simulink library "v2l"  (R2021b)
settings: Solver=VariableStepAuto  StartTime=0.0  StopTime=10.0  RelTol=1e-3
undefined symbols (not defined in the file): AV2L_SOCV2LLimit_X_pct, C_TASK_1000MS_S, ENUM_OBCV2LSTA_WORKING, ENUM_REQOBCEXTRV2L_EXTERNALDISCHRG, ENUM_REQOBCINTRV2L_INTERNALDISCHRG, ENUM_REQV2LIVIDISCHRG_DISCHRG, ENUM_REQV2LIVIDISCHRG_OFF, FALSE, KV2L_HVBattSOCLimit_pct, KV2L_HVPOGrpCheckOvrd_flg, KV2L_HVPOGrplowerLimit_pct, KV2L_HVPOGrpUpperLimit_pct, KV2L_OBCACCurrInfLimit_A, KV2L_SOCV2LSetLimit_pct, MV2L_SOCV2LLimit_Y_pct
libraries: hcu_lib x3, nmm x1, FVT_lib x1
settings Model: Creator=FVT23010  LastModifiedBy=FVT23010

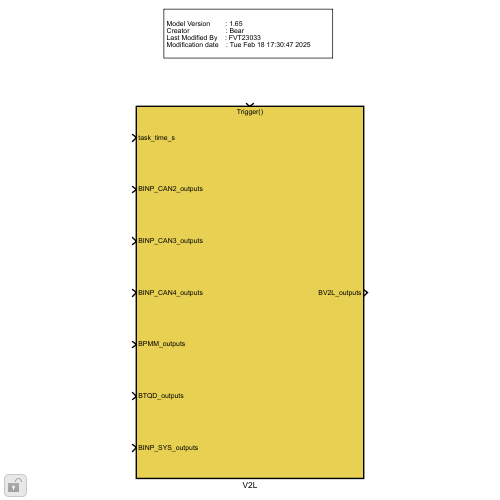
[thumbnail: Simulink's stored preview of the top-level diagram]
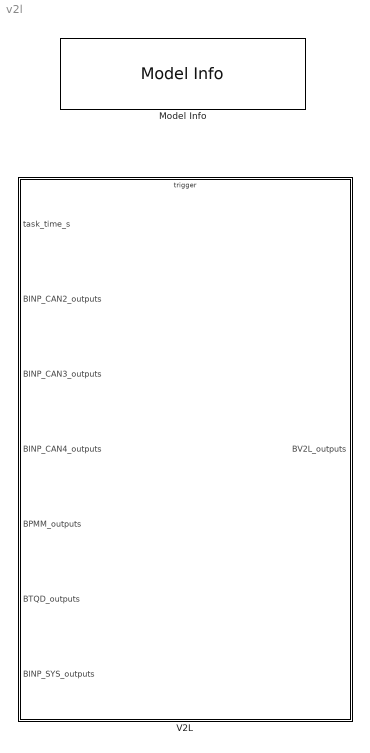
== system v2l ==
  Model Info : nmm/Model Info  InitialBlockCM=None  BlockCM=None  Frame=on  DisplayStringWithTags=|  HorizontalTextAlignment=Left  LeftAlignmentValue=0.02  SourceBlockDiagram=pmm  TagMaxNumber=20
      | Model Version        : %<ModelVersion>
      | Creator                   : Bear
      | Last Modified By    : %<LastModifiedBy>
      | Modification date    : %<LastModificationDate>
  V2L : Subsystem
      settings: RTWSystemCode=Nonreusable function  RTWFcnNameOpts=Use subsystem name  RTWFileNameOpts=Use subsystem name

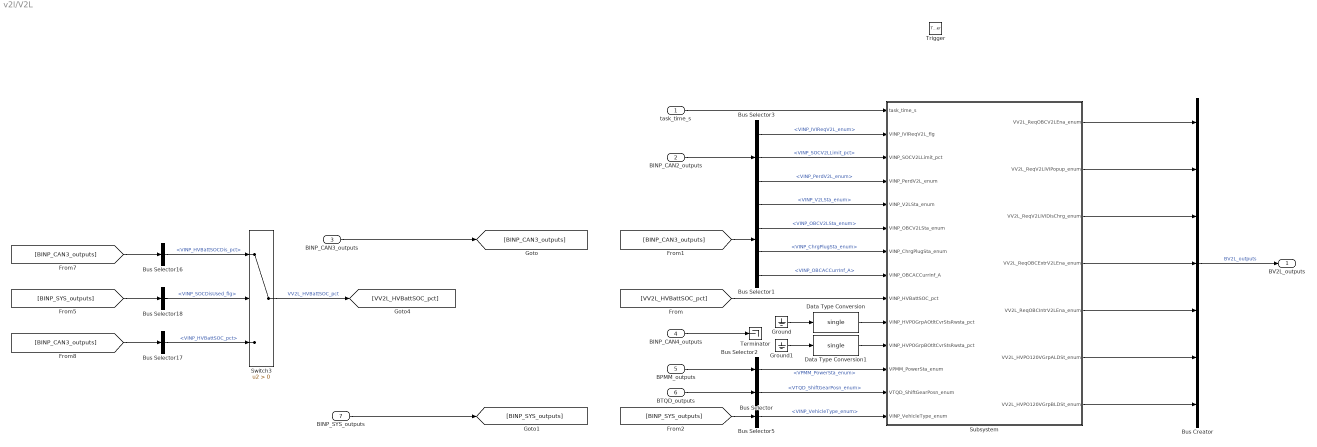
== system v2l/V2L ==
  task_time_s : Inport
  BINP_CAN2_outputs : Inport  Port=2  OutDataTypeStr=Bus: BINP_CAN2_outputs
  BINP_CAN3_outputs : Inport  Port=3  OutDataTypeStr=Bus: BINP_CAN3_outputs
  BINP_CAN4_outputs : Inport  Port=4  OutDataTypeStr=Bus: BINP_CAN4_outputs
  BPMM_outputs : Inport  Port=5  OutDataTypeStr=Bus: BPMM_outputs
  BTQD_outputs : Inport  Port=6  OutDataTypeStr=Bus: BTQD_outputs
  BINP_SYS_outputs : Inport  Port=7  OutDataTypeStr=Bus: BINP_SYS_outputs
  Trigger : TriggerPort  TriggerType=function-call  VariantControl=(inherit)  PortDimensions=1
  Bus Creator : BusCreator  Inputs=7  OutDataTypeStr=Bus: BV2L_outputs  NonVirtualBus=on
  Bus Selector : BusSelector  OutputSignals=VTQD_ShiftGearPosn_enum
  Bus Selector1 : BusSelector  OutputSignals=VINP_V2LSta_enum,VINP_OBCV2LSta_enum,VINP_ChrgPlugSta_enum,VINP_OBCACCurrInf_A
  Bus Selector16 : BusSelector  OutputSignals=VINP_HVBattSOCDis_pct
  Bus Selector17 : BusSelector  OutputSignals=VINP_HVBattSOC_pct
  Bus Selector18 : BusSelector  OutputSignals=VINP_SOCDisUsed_flg
  Bus Selector2 : BusSelector  OutputSignals=VPMM_PowerSta_enum
  Bus Selector3 : BusSelector  OutputSignals=VINP_IVIReqV2L_enum,VINP_SOCV2LLimit_pct,VINP_PerdV2L_enum
  Bus Selector5 : BusSelector  OutputSignals=VINP_VehicleType_enum
  Data Type Conversion : DataTypeConversion  OutDataTypeStr=single
  Data Type Conversion1 : DataTypeConversion  OutDataTypeStr=single
  Ground : Ground
  Ground1 : Ground
  Subsystem : Subsystem
  Switch3 : Switch  Criteria=u2 > Threshold
  Terminator : Terminator
  BV2L_outputs : Outport  OutDataTypeStr=Bus: BV2L_outputs
  wires:
  BPMM_outputs/1 -> Bus Selector2/1
  BTQD_outputs/1 -> Bus Selector/1
  BINP_CAN2_outputs/1 -> Bus Selector3/1
  Bus Creator/1 -> BV2L_outputs/1  "BV2L_outputs"
  Bus Selector3/1 -> Subsystem/2(VINP_IVIReqV2L_flg)  "<VINP_IVIReqV2L_enum>"
  Bus Selector3/2 -> Subsystem/3(VINP_SOCV2LLimit_pct)  "<VINP_SOCV2LLimit_pct>"
  Bus Selector3/3 -> Subsystem/4(VINP_PerdV2L_enum)  "<VINP_PerdV2L_enum>"
  Bus Selector1/1 -> Subsystem/5(VINP_V2LSta_enum)  "<VINP_V2LSta_enum>"
  Bus Selector1/2 -> Subsystem/6(VINP_OBCV2LSta_enum)  "<VINP_OBCV2LSta_enum>"
  Bus Selector1/3 -> Subsystem/7(VINP_ChrgPlugSta_enum)  "<VINP_ChrgPlugSta_enum>"
  Bus Selector1/4 -> Subsystem/8(VINP_OBCACCurrInf_A)  "<VINP_OBCACCurrInf_A>"
  Bus Selector2/1 -> Subsystem/12(VPMM_PowerSta_enum)  "<VPMM_PowerSta_enum>"
  Bus Selector/1 -> Subsystem/13(VTQD_ShiftGearPosn_enum)  "<VTQD_ShiftGearPosn_enum>"
  task_time_s/1 -> Subsystem/1(task_time_s)
  Subsystem/1(VV2L_ReqOBCV2LEna_enum) -> Bus Creator/1
  Subsystem/2(VV2L_ReqV2LIVIPopup_enum) -> Bus Creator/2
  Subsystem/3(VV2L_ReqV2LIVIDisChrg_enum) -> Bus Creator/3
  Subsystem/4(VV2L_ReqOBCExtrV2LEna_enum) -> Bus Creator/4
  Subsystem/5(VV2L_ReqOBCIntrV2LEna_enum) -> Bus Creator/5
  Subsystem/6(VV2L_HVPO120VGrpALDSt_enum) -> Bus Creator/6
  Subsystem/7(VV2L_HVPO120VGrpBLDSt_enum) -> Bus Creator/7
  Bus Selector5/1 -> Subsystem/14(VINP_VehicleType_enum)  "<VINP_VehicleType_enum>"
  Bus Selector16/1 -> Switch3/1  "<VINP_HVBattSOCDis_pct>"
  [BINP_CAN3_outputs] -> Bus Selector16/1
  [BINP_CAN3_outputs] -> Bus Selector17/1
  Switch3/1 -> [VV2L_HVBattSOC_pct]  "VV2L_HVBattSOC_pct"
  [BINP_SYS_outputs] -> Bus Selector18/1
  Bus Selector17/1 -> Switch3/3  "<VINP_HVBattSOC_pct>"
  Bus Selector18/1 -> Switch3/2  "<VINP_SOCDisUsed_flg>"
  [VV2L_HVBattSOC_pct] -> Subsystem/9(VINP_HVBattSOC_pct)
  BINP_CAN3_outputs/1 -> [BINP_CAN3_outputs]
  [BINP_CAN3_outputs] -> Bus Selector1/1
  BINP_SYS_outputs/1 -> [BINP_SYS_outputs]
  [BINP_SYS_outputs] -> Bus Selector5/1
  BINP_CAN4_outputs/1 -> Terminator/1
  Ground/1 -> Data Type Conversion/1
  Data Type Conversion/1 -> Subsystem/10(VINP_HVPOGrpAOtltCvrStsRwsta_pct)
  Ground1/1 -> Data Type Conversion1/1
  Data Type Conversion1/1 -> Subsystem/11(VINP_HVPOGrpBOtltCvrStsRwsta_pct)

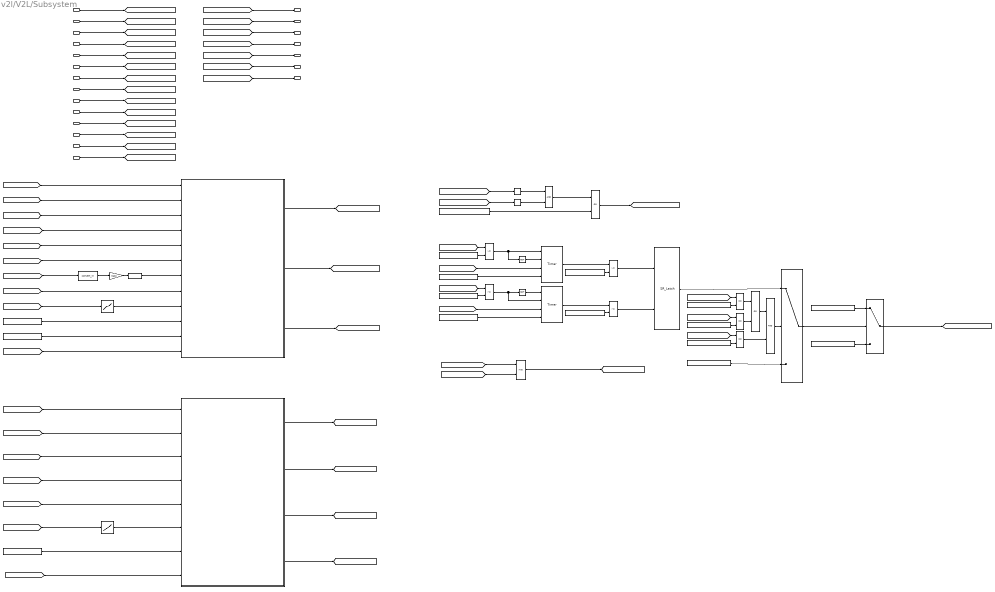
== system v2l/V2L/Subsystem ==
  task_time_s : Inport
  VINP_IVIReqV2L_flg : Inport  Port=2
  VINP_SOCV2LLimit_pct : Inport  Port=3
  VINP_PerdV2L_enum : Inport  Port=4
  VINP_V2LSta_enum : Inport  Port=5
  VINP_OBCV2LSta_enum : Inport  Port=6
  VINP_ChrgPlugSta_enum : Inport  Port=7
  VINP_OBCACCurrInf_A : Inport  Port=8
  VINP_HVBattSOC_pct : Inport  Port=9
  VINP_HVPOGrpAOtltCvrStsRwsta_pct : Inport  Port=10
  VINP_HVPOGrpBOtltCvrStsRwsta_pct : Inport  Port=11
  VPMM_PowerSta_enum : Inport  Port=12
  VTQD_ShiftGearPosn_enum : Inport  Port=13
  VINP_VehicleType_enum : Inport  Port=14
  1-D Lookup Table : Lookup_n-D  NumberOfTableDimensions=1  BreakpointsForDimension1=AV2L_SOCV2LLimit_X_pct  Table=MV2L_SOCV2LLimit_Y_pct  InternalRulePriority=Speed  RndMeth=Simplest  InputSameDT=on
  1-D Lookup Table1 : Lookup_n-D  NumberOfTableDimensions=1  BreakpointsForDimension1=AV2L_SOCV2LLimit_X_pct  Table=MV2L_SOCV2LLimit_Y_pct  InternalRulePriority=Speed  RndMeth=Simplest  InputSameDT=on
  Constant : Constant  Value=KV2L_HVBattSOCLimit_pct
  Constant1 : Constant  Value=KV2L_SOCV2LSetLimit_pct
  Constant10 : Constant  Value=ENUM_REQV2LIVIDISCHRG_OFF
  Constant11 : Constant  Value=ENUM_REQV2LIVIDISCHRG_DISCHRG
  Constant12 : Constant  Value=ENUM_REQOBCEXTRV2L_EXTERNALDISCHRG
  Constant13 : Constant  Value=ENUM_REQOBCINTRV2L_INTERNALDISCHRG
  Constant14 : Constant  Value=KV2L_HVPOGrpCheckOvrd_flg
  Constant15 : Constant  Value=ENUM_OBCV2LSTA_WORKING
  Constant2 : Constant  Value=KV2L_HVBattSOCLimit_pct
  Constant3 : Constant  Value=KV2L_OBCACCurrInfLimit_A
  Constant{4..5,7..8} (4 alike) : Constant  Value=C_TASK_1000MS_S
  Constant6 : Constant  Value=KV2L_OBCACCurrInfLimit_A
  Constant9 : Constant  Value=FALSE
  Data Type Conversion : DataTypeConversion  OutDataTypeStr=single
  External V2L : Stateflow chart  TreatAsAtomicUnit=on
      settings: PortSchema="{\"entries\":[{\"content\":{\"sides\":[{\"content\":{\"connectorIds\":[\"In1\",\"In2\",\"In3\",\"In4\",\"In5\",\"In6\",\"In7\",\"In8\",\"In9\",\"In10\",\"In11\",\"In12\"]},\"type\":\"ConnectorPlacement.EquallySpacedRectSide\",\"uuid\":\"45116e41-1dba-4e2c-ae04-6007bf1e0ef0\"},{\"content\":{\"connectorIds\":[\"Out1\",\"Out3\",\"Out2\"],\"side\":\"RIGHT\"},\"type\":\"ConnectorPlacement.EquallySpacedRectSide\",\"uuid\":\"1413f850-bb59-4483-bd31-f1fc97818d70\"},{\"content\":{\"connectorIds\":[],\"side\":\"TOP\"},\"type\":\"ConnectorPlacement.EquallySpacedRectSide\",\"uuid\":\"54439ff1-b412-4fc1-ba32-699466081697\"}]},\"type\":\"ConnectorPlacement.EquallySpacedConnector\",\"uuid\":\"a2cf914b-1bae-4478-a72c-e2494d61996c\"}],\"packageUris\":[\"http://schema.mathworks.com/mf0/Connector/R2020b\"],\"version\":\"1.0\"}"
  Gain : Gain  Gain=3600
  Internal V2L : Stateflow chart  TreatAsAtomicUnit=on
  Logical Operator : Logic  AllPortsSameDT=off  OutDataTypeStr=boolean
  Logical Operator1 : Logic  Operator=NOT  AllPortsSameDT=off  OutDataTypeStr=boolean
  Logical Operator2 : Logic  Operator=NOT  AllPortsSameDT=off  OutDataTypeStr=boolean
  Logical Operator3 : Logic  Operator=OR  AllPortsSameDT=off  OutDataTypeStr=boolean
  Logical Operator4 : Logic  AllPortsSameDT=off  OutDataTypeStr=boolean
  Logical Operator5 : Logic  Operator=OR  AllPortsSameDT=off  OutDataTypeStr=boolean
  MinMax : MinMax  Function=max  Inputs=2
  Relational Operator{,1..3} (4 alike) : RelationalOperator  OutDataTypeStr=boolean  RndMeth=Simplest
  Relational Operator4 : RelationalOperator  Operator===  OutDataTypeStr=boolean  RndMeth=Simplest
  Relational Operator5 : RelationalOperator  Operator===  OutDataTypeStr=boolean  RndMeth=Simplest
  Relational Operator6 : RelationalOperator  Operator===  OutDataTypeStr=boolean  RndMeth=Simplest
  Relay : Relay  OnSwitchValue=KV2L_HVPOGrpUpperLimit_pct  OffSwitchValue=KV2L_HVPOGrplowerLimit_pct
  Relay1 : Relay  OnSwitchValue=KV2L_HVPOGrpUpperLimit_pct  OffSwitchValue=KV2L_HVPOGrplowerLimit_pct
  SR_Latch : hcu_lib/Basic_Blocks/SR_Latch
  Switch : Switch  Criteria=u2 ~= 0
  Switch1 : Switch  Criteria=u2 ~= 0
  Timer : hcu_lib/Basic_Blocks/Timer
  Timer1 : hcu_lib/Basic_Blocks/Timer
  convert_in9 : FVT_lib/hal/convert_in  gain=0.5  offset=0.5
  VV2L_ReqOBCV2LEna_enum : Outport
  VV2L_ReqV2LIVIPopup_enum : Outport  Port=2
  VV2L_ReqV2LIVIDisChrg_enum : Outport  Port=3
  VV2L_ReqOBCExtrV2LEna_enum : Outport  Port=4
  VV2L_ReqOBCIntrV2LEna_enum : Outport  Port=5
  VV2L_HVPO120VGrpALDSt_enum : Outport  Port=6
  VV2L_HVPO120VGrpBLDSt_enum : Outport  Port=7
  wires:
  task_time_s/1 -> [task_time_s]
  [VV2L_ReqOBCExtrV2LEna_enum] -> VV2L_ReqOBCExtrV2LEna_enum/1
  [task_time_s] -> External V2L/1(task_time_s)
  Constant1/1 -> External V2L/11(KV2L_SOCV2LSetLimit_pct)
  External V2L/1(VV2L_ReqOBCExtrV2LEna_enum) -> [VV2L_ReqOBCExtrV2LEna_enum]
  VTQD_ShiftGearPosn_enum/1 -> [VTQD_ShiftGearPosn_enum]
  VINP_IVIReqV2L_flg/1 -> [VINP_IVIReqV2L_flg]
  VINP_SOCV2LLimit_pct/1 -> [VINP_SOCV2LLimit_pct]
  VINP_V2LSta_enum/1 -> [VINP_V2LSta_enum]
  VINP_OBCV2LSta_enum/1 -> [VINP_OBCV2LSta_enum]
  [VINP_HVBattSOC_pct] -> External V2L/6(VINP_HVBattSOC_pct)
  VINP_PerdV2L_enum/1 -> [VINP_PerdV2L_enum]
  [VINP_SOCV2LLimit_pct] -> 1-D Lookup Table/1
  VPMM_PowerSta_enum/1 -> [VPMM_PowerSta_enum]
  [VINP_IVIReqV2L_flg] -> External V2L/2(VINP_IVIReqV2L_flg)
  [VINP_V2LSta_enum] -> External V2L/5(VINP_V2LSta_enum)
  [VINP_OBCV2LSta_enum] -> External V2L/8(VINP_OBCV2LSta_enum)
  VINP_HVBattSOC_pct/1 -> [VINP_HVBattSOC_pct]
  [VPMM_PowerSta_enum] -> External V2L/3(VPMM_PowerSta_enum)
  Constant/1 -> External V2L/10(KV2L_HVBattSOCLimit_pct)
  [VV2L_ReqV2LIVIPopup_enum] -> VV2L_ReqV2LIVIPopup_enum/1
  [VTQD_ShiftGearPosn_enum] -> External V2L/4(VTQD_ShiftGearPosn_enum)
  Data Type Conversion/1 -> External V2L/7(VV2L_PerdV2LSet_s)  "VV2L_PerdV2LSet_s"
  Gain/1 -> Data Type Conversion/1
  [VINP_PerdV2L_enum] -> convert_in9/1
  convert_in9/1 -> Gain/1
  1-D Lookup Table/1 -> External V2L/9(VV2L_SOCV2LLimit_pct)  "VV2L_SOCV2LLimit_pct"
  Constant2/1 -> Internal V2L/7(KV2L_HVBattSOCLimit_pct)
  [VPMM_PowerSta_enum] -> Internal V2L/3(VPMM_PowerSta_enum)
  [VINP_OBCV2LSta_enum] -> Internal V2L/5(VINP_OBCV2LSta_enum)
  [VINP_SOCV2LLimit_pct] -> 1-D Lookup Table1/1
  [VINP_HVBattSOC_pct] -> Internal V2L/4(VINP_HVBattSOC_pct)
  VINP_ChrgPlugSta_enum/1 -> [VINP_ChrgPlugSta_enum]
  [VINP_ChrgPlugSta_enum] -> Internal V2L/1(VINP_ChrgPlugSta_enum)
  [VINP_HVPOGrpAOtltCvrStsRwsta_pct] -> Relay/1
  [VINP_HVPOGrpBOtltCvrStsRwsta_pct] -> Relay1/1
  Relay/1 -> Logical Operator/1
  Relay1/1 -> Logical Operator/2
  Logical Operator/1 -> Logical Operator5/1
  [VV2L_HVPOGrpCheck_flg] -> Internal V2L/2(VV2L_HVPOGrpCheck_flg)
  VINP_OBCACCurrInf_A/1 -> [VINP_OBCACCurrInf_A]
  [VINP_OBCACCurrInf_A] -> Relational Operator/1
  Constant3/1 -> Relational Operator/2
  Relational Operator/1 -> Logical Operator1/1, Timer/1
  Logical Operator1/1 -> Timer/2
  [task_time_s] -> Timer/3
  Constant4/1 -> Timer/4
  Timer/1 -> Relational Operator1/1
  Constant5/1 -> Relational Operator1/2
  Relational Operator1/1 -> SR_Latch/1
  Relational Operator3/1 -> SR_Latch/2
  Constant8/1 -> Relational Operator3/2
  Timer1/1 -> Relational Operator3/1
  Constant7/1 -> Timer1/4
  [task_time_s] -> Timer1/3
  Relational Operator2/1 -> Timer1/2, Logical Operator2/1
  Constant6/1 -> Relational Operator2/2
  [VINP_OBCACCurrInf_A] -> Relational Operator2/1
  Logical Operator2/1 -> Timer1/1
  SR_Latch/1 -> Switch/1
  Internal V2L/1(VV2L_ReqOBCIntrV2LEna_enum) -> [VV2L_ReqOBCIntrV2LEna_enum]
  [VV2L_ReqExtrV2LIVIPopup_enum] -> MinMax/1
  Internal V2L/4(VV2L_ReqIntrV2LIVIPopup_enum) -> [VV2L_ReqIntrV2LIVIPopup_enum]
  [VV2L_ReqIntrV2LIVIPopup_enum] -> MinMax/2
  MinMax/1 -> [VV2L_ReqV2LIVIPopup_enum]  "VV2L_ReqV2LIVIPopup_enum"
  Switch/1 -> Switch1/2
  [VV2L_ReqOBCExtrV2LEna_enum] -> Relational Operator4/1
  [VV2L_ReqOBCIntrV2LEna_enum] -> Relational Operator5/1
  Logical Operator3/1 -> Logical Operator4/1
  Constant9/1 -> Switch/3
  Internal V2L/3(VV2L_HVPO120VGrpBLDSt_enum) -> [VV2L_HVPO120VGrpBLDSt_enum]
  Internal V2L/2(VV2L_HVPO120VGrpALDSt_enum) -> [VV2L_HVPO120VGrpALDSt_enum]
  1-D Lookup Table1/1 -> Internal V2L/6(VV2L_SOCV2LLimit_pct)  "VV2L_SOCV2LLimit_pct"
  [VV2L_ReqOBCIntrV2LEna_enum] -> VV2L_ReqOBCIntrV2LEna_enum/1
  [VV2L_ReqV2LIVIDisChrg_enum] -> VV2L_ReqV2LIVIDisChrg_enum/1
  [VV2L_HVPO120VGrpALDSt_enum] -> VV2L_HVPO120VGrpALDSt_enum/1
  [VV2L_HVPO120VGrpBLDSt_enum] -> VV2L_HVPO120VGrpBLDSt_enum/1
  VINP_HVPOGrpAOtltCvrStsRwsta_pct/1 -> [VINP_HVPOGrpAOtltCvrStsRwsta_pct]
  VINP_HVPOGrpBOtltCvrStsRwsta_pct/1 -> [VINP_HVPOGrpBOtltCvrStsRwsta_pct]
  [VV2L_ReqOBCV2LEna_enum] -> VV2L_ReqOBCV2LEna_enum/1
  External V2L/2(VV2L_ReqExtrV2LIVIPopup_enum) -> [VV2L_ReqExtrV2LIVIPopup_enum]
  External V2L/3(VV2L_ReqOBCV2LEna_enum) -> [VV2L_ReqOBCV2LEna_enum]
  Constant10/1 -> Switch1/3
  Constant11/1 -> Switch1/1
  Switch1/1 -> [VV2L_ReqV2LIVIDisChrg_enum]  "VV2L_ReqV2LIVIDisChrg_enum"
  Logical Operator4/1 -> Switch/2
  [VINP_OBCV2LSta_enum] -> Relational Operator6/1
  Relational Operator4/1 -> Logical Operator3/1
  Relational Operator5/1 -> Logical Operator3/2
  Constant12/1 -> Relational Operator4/2
  Constant13/1 -> Relational Operator5/2
  Logical Operator5/1 -> [VV2L_HVPOGrpCheck_flg]  "VV2L_HVPOGrpCheck_flg"
  Constant14/1 -> Logical Operator5/2
  VINP_VehicleType_enum/1 -> [VINP_VehicleType_enum]
  [VINP_VehicleType_enum] -> Internal V2L/8(VINP_VehicleType_enum)
  [VINP_VehicleType_enum] -> External V2L/12(VINP_VehicleType_enum)
  Constant15/1 -> Relational Operator6/2
  Relational Operator6/1 -> Logical Operator4/2

== stateflow chart v2l/V2L/Subsystem/Internal V2L ==
  state V2L
    en:
    VV2L_ReqOBCIntrV2LEna_enum = ENUM_REQOBCINTRV2L_NOREQUEST;
    VV2L_ReqIntrV2LIVIPopup_enum = ENUM_REQV2LIVI_NOREQUEST;
    VV2L_HVPO120VGrpALDSt_enum = ENUM_HVPO120VGRPDST_OFF;
    VV2L_HVPO120VGrpBLDSt_enum = ENUM_HVPO120VGRPDST_OFF;
    % 第一版先不考慮V2L放電模式下，更改設定時間的可能
    (default) -> (junction 102)
    V2L -> (junction 102) : {VV2L_ReqIntrV2LIVIPopup_enum = ENUM_REQV2LIVI_NOREQUEST}
    (junction 102) -> (junction 268) [order 1] : [VINP_VehicleType_enum == ENUM_VEHICLETYPE_D31F25 || ...
        | VINP_VehicleType_enum == ENUM_VEHICLETYPE_D31HRWD || ...
        | VINP_VehicleType_enum == ENUM_VEHICLETYPE_D31HAWD]
    (junction 268) -> (junction 240) [order 1] : [VINP_ChrgPlugSta_enum == ENUM_CHRGPLUGSTA_NONE]
    (junction 240) -> (junction 16) [order 1] : [(VPMM_PowerSta_enum == ENUM_POWERSTA_ON || VPMM_PowerSta_enum == ENUM_POWERSTA_READY) && ...
        | VV2L_HVPOGrpCheck_flg]
    (junction 16) -> (junction 45) [order 1] : [VINP_HVBattSOC_pct > KV2L_HVBattSOCLimit_pct]
    (junction 45) -> (junction 59) [order 1] : [VINP_HVBattSOC_pct > VV2L_SOCV2LLimit_pct]
    (junction 59) -> (junction 61) [order 1] : [VINP_OBCV2LSta_enum == ENUM_OBCV2LSTA_FAULT]
    (junction 102) -> (junction 108) [order 2]
    (junction 268) -> (junction 269) [order 2] : {VV2L_ReqIntrV2LIVIPopup_enum = ENUM_REQV2LIVI_STOPBYPLUG;}
    (junction 240) -> (junction 242) [order 2]
    (junction 16) -> (junction 200) [order 2] : {VV2L_ReqIntrV2LIVIPopup_enum = ENUM_REQV2LIVI_SOCTOOLOW;}
    (junction 45) -> (junction 203) [order 2] : {VV2L_ReqIntrV2LIVIPopup_enum = ENUM_REQV2LIVI_STOPBYSOC;}
    (junction 59) -> (junction 218) [order 2] : {
        | VV2L_ReqOBCIntrV2LEna_enum = ENUM_REQOBCINTRV2L_INTERNALDISCHRG;
        | }
    (junction 61) -> (junction 63) : {VV2L_ReqIntrV2LIVIPopup_enum = ENUM_REQV2LIVI_FAULT;}
    (junction 218) -> (junction 261) [order 1] : [VINP_OBCV2LSta_enum == ENUM_OBCV2LSTA_WORKING]
    (junction 218) -> (junction 262) [order 2] : {
        | VV2L_HVPO120VGrpALDSt_enum = ENUM_HVPO120VGRPDST_OFF;
        | VV2L_HVPO120VGrpBLDSt_enum  = ENUM_HVPO120VGRPDST_OFF;
        | }
    (junction 261) -> (junction 263) : {
        | VV2L_HVPO120VGrpALDSt_enum = ENUM_HVPO120VGRPDST_GREEN;
        | VV2L_HVPO120VGrpBLDSt_enum  = ENUM_HVPO120VGRPDST_GREEN;
        | }
    (junction 269) -> (junction 242)
    (junction 242) -> (junction 200)
    (junction 200) -> (junction 203)
    (junction 203) -> (junction 63)
    (junction 108) -> (junction 269)
    (junction 63) -> (junction 196) : {VV2L_ReqOBCIntrV2LEna_enum = ENUM_REQOBCINTRV2L_NOREQUEST;
        | VV2L_HVPO120VGrpALDSt_enum = ENUM_HVPO120VGRPDST_OFF;
        | VV2L_HVPO120VGrpBLDSt_enum = ENUM_HVPO120VGRPDST_OFF;}
  (default) -> V2L
  data: VINP_ChrgPlugSta_enum input; VV2L_HVPOGrpCheck_flg input; VPMM_PowerSta_enum input; VINP_HVBattSOC_pct input; VV2L_ReqOBCIntrV2LEna_enum output uint8; ENUM_POWERSTA_ON parameter; ENUM_REQV2LIVI_SOCTOOLOW parameter; ENUM_REQV2LIVI_FAULT parameter; VINP_OBCV2LSta_enum input; ENUM_OBCV2LSTA_FAULT parameter; VV2L_SOCV2LLimit_pct input; ENUM_REQV2LIVI_NOREQUEST parameter; ENUM_REQV2LIVI_STOPBYSOC parameter; KV2L_HVBattSOCLimit_pct input; VV2L_HVPO120VGrpALDSt_enum output double; VV2L_HVPO120VGrpBLDSt_enum output double; ENUM_CHRGPLUGSTA_NONE parameter; ENUM_HVPO120VGRPDST_GREEN parameter; ENUM_HVPO120VGRPDST_OFF parameter; ENUM_POWERSTA_READY parameter; ENUM_REQV2LIVI_STOPBYPLUG parameter; VV2L_ReqIntrV2LIVIPopup_enum output double; ENUM_REQOBCINTRV2L_INTERNALDISCHRG parameter; ENUM_REQOBCINTRV2L_NOREQUEST parameter; ENUM_OBCV2LSTA_WORKING parameter; VINP_VehicleType_enum input; ENUM_VEHICLETYPE_D31F25 parameter; ENUM_VEHICLETYPE_D31HAWD parameter; ENUM_VEHICLETYPE_D31HRWD parameter

== stateflow chart v2l/V2L/Subsystem/External V2L ==
  state V2L
    en:
    VV2L_PerdV2LTimer_s = 0;
    VV2L_ReqOBCV2LEna_enum = ENUM_REQOBCV2L_NOREQUEST;
    VV2L_ReqOBCExtrV2LEna_enum = ENUM_REQOBCEXTRV2L_NOREQUEST;
    VV2L_ReqExtrV2LIVIPopup_enum = ENUM_REQV2LIVI_NOREQUEST;
    % 第一版先不考慮V2L放電模式下，更改設定時間的可能
    (default) -> (junction 102)
    V2L -> (junction 102) : {VV2L_ReqExtrV2LIVIPopup_enum = ENUM_REQV2LIVI_NOREQUEST}
    (junction 102) -> (junction 16) [order 1] : [VINP_IVIReqV2L_flg]
    (junction 16) -> (junction 191) [order 1] : [VINP_HVBattSOC_pct > KV2L_HVBattSOCLimit_pct]
    (junction 191) -> (junction 45) [order 1] : [VV2L_SOCV2LLimit_pct >= KV2L_SOCV2LSetLimit_pct]
    (junction 45) -> (junction 53) [order 1] : [VINP_HVBattSOC_pct > VV2L_SOCV2LLimit_pct]
    (junction 53) -> (junction 168) [order 1] : [VV2L_PerdV2LSet_s > VV2L_PerdV2LTimer_s]
        | {VV2L_PerdV2LTimer_s += task_time_s;}
    (junction 168) -> (junction 217) [order 1] : [VTQD_ShiftGearPosn_enum == ENUM_GEARPOSNTOCAN_P && VPMM_PowerSta_enum == ENUM_POWERSTA_ON]
    (junction 217) -> (junction 180) [order 1] : [VINP_V2LSta_enum == ENUM_V2LSTA_PLUGIN || VINP_V2LSta_enum == ENUM_V2LSTA_SWON]
    (junction 180) -> (junction 59) [order 1] : [VINP_V2LSta_enum == ENUM_V2LSTA_SWON]
    (junction 59) -> (junction 61) [order 1] : [VINP_OBCV2LSta_enum == ENUM_OBCV2LSTA_FAULT]
    (junction 102) -> (junction 108) [order 2]
    (junction 16) -> (junction 200) [order 2] : {VV2L_ReqExtrV2LIVIPopup_enum = ENUM_REQV2LIVI_SOCTOOLOW;}
    (junction 191) -> (junction 192) [order 2]
    (junction 45) -> (junction 203) [order 2] : {VV2L_ReqExtrV2LIVIPopup_enum = ENUM_REQV2LIVI_STOPBYSOC;}
    (junction 53) -> (junction 205) [order 2] : {VV2L_ReqExtrV2LIVIPopup_enum = ENUM_REQV2LIVI_TIMEUP;}
    (junction 168) -> (junction 257) [order 2]
    (junction 217) -> (junction 223) [order 2]
    (junction 180) -> (junction 226) [order 2] : {VV2L_ReqExtrV2LIVIPopup_enum = ENUM_REQV2LIVI_PLUGINSWOFF;
        | VV2L_ReqOBCExtrV2LEna_enum = ENUM_REQOBCEXTRV2L_NOREQUEST;
        | VV2L_ReqOBCV2LEna_enum = ENUM_REQOBCV2L_NOREQUEST;
        | VV2L_PerdV2LTimer_s = 0;}
    (junction 59) -> (junction 218) [order 2] : {
        | VV2L_ReqOBCV2LEna_enum= ENUM_REQOBCV2L_EXTERNALDISCHRG;
        | }
    (junction 61) -> (junction 63) : {VV2L_ReqExtrV2LIVIPopup_enum = ENUM_REQV2LIVI_FAULT;}
    (junction 218) -> (junction 243) [order 1] : [VINP_VehicleType_enum == ENUM_VEHICLETYPE_D31F25 || ...
        | VINP_VehicleType_enum == ENUM_VEHICLETYPE_D31HRWD || ...
        | VINP_VehicleType_enum == ENUM_VEHICLETYPE_D31HAWD]
    (junction 218) -> (junction 244) [order 2] : {
        | VV2L_ReqOBCExtrV2LEna_enum = ENUM_REQOBCEXTRV2L_NOREQUEST;
        | }
    (junction 243) -> (junction 245) : {
        | VV2L_ReqOBCExtrV2LEna_enum = ENUM_REQOBCEXTRV2L_EXTERNALDISCHRG;
        | }
    (junction 257) -> (junction 253) [order 1] : [VINP_V2LSta_enum != ENUM_V2LSTA_NOPLUG && ...
        | (VINP_VehicleType_enum ==ENUM_VEHICLETYPE_D31L24 ||...
        | VINP_VehicleType_enum ==ENUM_VEHICLETYPE_D21)]
    (junction 257) -> (junction 207) [order 2]
    (junction 253) -> (junction 259) : {VV2L_ReqExtrV2LIVIPopup_enum = ENUM_REQV2LIVI_CHECKPLUG;}
    (junction 108) -> (junction 200)
    (junction 200) -> (junction 192)
    (junction 192) -> (junction 203)
    (junction 203) -> (junction 205)
    (junction 205) -> (junction 207)
    (junction 207) -> (junction 259)
    (junction 259) -> (junction 223)
    (junction 223) -> (junction 63)
    (junction 63) -> (junction 196) : {VV2L_ReqOBCExtrV2LEna_enum = ENUM_REQOBCEXTRV2L_NOREQUEST;
        | VV2L_ReqOBCV2LEna_enum = ENUM_REQOBCV2L_NOREQUEST;
        | VV2L_PerdV2LTimer_s = 0;}
  (default) -> V2L
  data: task_time_s input; VINP_IVIReqV2L_flg input; VPMM_PowerSta_enum input; VTQD_ShiftGearPosn_enum input; VINP_V2LSta_enum input; VINP_HVBattSOC_pct input; VV2L_PerdV2LSet_s input; VV2L_ReqOBCExtrV2LEna_enum output uint8; ENUM_GEARPOSNTOCAN_P parameter; ENUM_POWERSTA_ON parameter; ENUM_V2LSTA_PLUGIN parameter; ENUM_V2LSTA_SWON parameter; ENUM_REQV2LIVI_SOCTOOLOW parameter; ENUM_REQV2LIVI_FAULT parameter; ENUM_REQV2LIVI_TIMEUP parameter; ENUM_REQV2LIVI_PLUGINSWOFF parameter; VINP_OBCV2LSta_enum input; VV2L_PerdV2LTimer_s local double; ENUM_OBCV2LSTA_FAULT parameter; VV2L_SOCV2LLimit_pct input; ENUM_REQV2LIVI_NOREQUEST parameter; ENUM_REQV2LIVI_STOPBYSOC parameter; KV2L_HVBattSOCLimit_pct input; KV2L_SOCV2LSetLimit_pct input; ENUM_REQOBCV2L_EXTERNALDISCHRG parameter; ENUM_REQOBCV2L_NOREQUEST parameter; VV2L_ReqExtrV2LIVIPopup_enum output double; VV2L_ReqOBCV2LEna_enum output double; ENUM_REQOBCEXTRV2L_EXTERNALDISCHRG parameter; ENUM_REQOBCEXTRV2L_NOREQUEST parameter; VINP_VehicleType_enum input; ENUM_VEHICLETYPE_D31F25 parameter; ENUM_VEHICLETYPE_D31HAWD parameter; ENUM_VEHICLETYPE_D31HRWD parameter; ENUM_REQV2LIVI_CHECKPLUG parameter; ENUM_V2LSTA_NOPLUG parameter; ENUM_VEHICLETYPE_D21 parameter; ENUM_VEHICLETYPE_D31L24 parameter
